simulink model "modele"  (R2025b)
settings: Solver=VariableStepAuto  StartTime=0.0  StopTime=10  RelTol=1e-3
values from neighbouring files (symbols this model uses):
  A = [0            0        1            0 ... (first row only)    [zad1.m]
  B = [c1/m1 ... (first row only)    [zad1.m]
  C = [1 0 0 0]    [zad1.m]
  c1 = 100    [zad1.m]
  c2 = 2000    [zad1.m]
  D = 0    [zad1.m]
  k1 = 370000    [zad1.m]
  k2 = 35000    [zad1.m]
  m1 = 90    [zad1.m]
  m2 = 600    [zad1.m]
undefined symbols (not defined in the file or in its folder): den, num
libraries: SignalEditorBlockLib x1
settings Model: Creator=D106-Student  LastModifiedBy=kubam

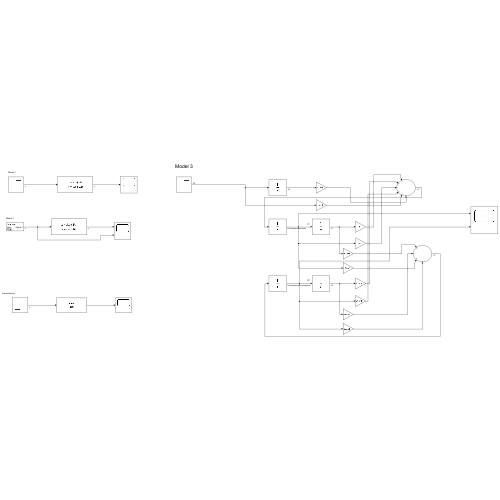
[thumbnail: Simulink's stored preview of the top-level diagram]
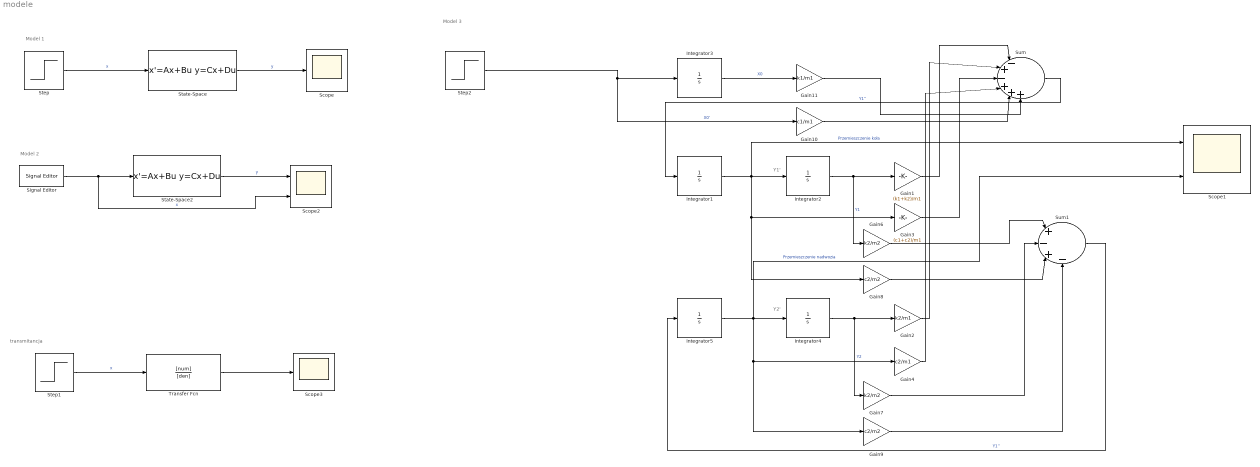
== system modele ==
  note: transmitancja
  note: Y1'
  note: Model 2
  note: Y2'
  note: Model 1
  note: Model 3
  Gain1 : Gain  Gain=(k1+k2)/m1
  Gain10 : Gain  Gain=c1/m1
  Gain11 : Gain  Gain=k1/m1
  Gain2 : Gain  Gain=k2/m1
  Gain3 : Gain  Gain=(c1+c2)/m1
  Gain4 : Gain  Gain=c2/m1
  Gain6 : Gain  Gain=k2/m2
  Gain7 : Gain  Gain=k2/m2
  Gain8 : Gain  Gain=c2/m2
  Gain9 : Gain  Gain=c2/m2
  Integrator{1..5} (5 alike) : Integrator
  Scope : Scope
      settings: ActiveDisplayYMinimum=-0.6831757999390633  ActiveDisplayYMaximum=2.7332835079922719
  Scope1 : Scope  NumInputPorts=2
      settings: ActiveDisplayYMinimum=-960.34288063558085  ActiveDisplayYMaximum=952.70179217502346
  Scope2 : Scope  NumInputPorts=2
      settings: ActiveDisplayYMinimum=-0.20887906055992805  ActiveDisplayYMaximum=0.27641423288631312  DataLoggingVariableName=ScopeData2
  Scope3 : Scope
      settings: ActiveDisplayYMinimum=-0.24159665316042744  ActiveDisplayYMaximum=1.858268215922855  DataLoggingVariableName=ScopeData3
  Signal Editor : SignalEditorBlockLib/Signal Editor  FileName=nierownosci.mat  ActiveScenario=Scenario  ActiveSignal=Signal 1  IsBus=off  OutputBusObjectStr=Bus: BusObject  SampleTime=0  ZeroCross=off  OutputAfterFinalValue=Setting to zero  Unit=inherit  PreserveSignalName=on  ApplySigPropsToAllScenarios=on  ApplySigPropsToAllSignals=off  SignalPropertySource=Dialog parameters
  State-Space : StateSpace  A=A  B=B  C=C  D=D  InitialCondition=0  ContinuousStateAttributes="\"position\""
  State-Space2 : StateSpace  A=A  B=B  C=C  D=D  InitialCondition=0  ContinuousStateAttributes="\"position\""
  Step : Step  SampleTime=0
  Step1 : Step  SampleTime=0
  Step2 : Step  SampleTime=0
  Sum : Sum  Inputs=|-+-+++
  Sum1 : Sum  Inputs=|+-+-
  Transfer Fcn : TransferFcn  Numerator=[num]  Denominator=[den]
  wires:
  Step/1 -> State-Space/1  "x"
  State-Space/1 -> Scope/1  "y"
  Signal Editor/1 -> Scope2/2, State-Space2/1  "x"
  State-Space2/1 -> Scope2/1  "y"
  Step2/1 -> Gain10/1, Integrator3/1  "X0'"
  Integrator1/1 -> Scope1/1, Gain8/1, Gain3/1, Integrator2/1  "Przemieszczenie koła"
  Integrator2/1 -> Gain6/1, Gain1/1  "Y1"
  Integrator5/1 -> Scope1/2, Integrator4/1, Gain9/1, Gain4/1  "Przemieszczenie nadwozia"
  Integrator4/1 -> Gain7/1, Gain2/1  "Y2"
  Sum/1 -> Integrator1/1  "Y1''"
  Gain6/1 -> Sum1/1
  Gain7/1 -> Sum1/2
  Gain8/1 -> Sum1/3
  Gain9/1 -> Sum1/4
  Sum1/1 -> Integrator5/1  "Y1''"
  Gain1/1 -> Sum/1
  Gain2/1 -> Sum/2
  Gain3/1 -> Sum/3
  Gain4/1 -> Sum/4
  Gain11/1 -> Sum/6
  Integrator3/1 -> Gain11/1  "X0"
  Gain10/1 -> Sum/5
  Step1/1 -> Transfer Fcn/1  "x"
  Transfer Fcn/1 -> Scope3/1
